simulink model "RL_sus_quarter_sim"  (R2025a)
settings: Solver=FixedStepAuto  StartTime=0.0  StopTime=20  FixedStep=0.001  RelTol=1e-3
model workspace (MAT data in the model file):
  G0 : Simulink.Parameter (value not decoded)
  Q_F : Simulink.Parameter (value not decoded)
  Q_dot_s : Simulink.Parameter (value not decoded)
  Q_dot_s_h : Simulink.Parameter (value not decoded)
  Q_dot_u : Simulink.Parameter (value not decoded)
  Q_flec : Simulink.Parameter (value not decoded)
  Q_flec_t : Simulink.Parameter (value not decoded)
  b_deflec : Simulink.Parameter (value not decoded)
  bump_height : Simulink.Parameter (value not decoded)
  bump_lenth : Simulink.Parameter (value not decoded)
  bump_start : Simulink.Parameter (value not decoded)
  f0 : Simulink.Parameter (value not decoded)
  kt : Simulink.Parameter (value not decoded)
  ms : Simulink.Parameter (value not decoded)
  n0 : Simulink.Parameter (value not decoded)
  n1 : Simulink.Parameter (value not decoded)
  omega_1 : Simulink.Parameter (value not decoded)
  omega_2 : Simulink.Parameter (value not decoded)
  omega_3 : Simulink.Parameter (value not decoded)
  omega_4 : Simulink.Parameter (value not decoded)
  ramp_height : Simulink.Parameter (value not decoded)
  ramp_lenth : Simulink.Parameter (value not decoded)
  ramp_start : Simulink.Parameter (value not decoded)
  sine_amp : Simulink.Parameter (value not decoded)
  sine_freq : Simulink.Parameter (value not decoded)
  u : Simulink.Parameter (value not decoded)
symbols that are objects in the model workspace (value not decoded): b_deflec, bump_height, bump_lenth, bump_start, f0, G0, kt, ms, n0, n1, omega_1, omega_2, omega_3, omega_4, Q_dot_s, Q_dot_s_h, Q_F, Q_flec, Q_flec_t, ramp_height, ramp_lenth, ramp_start, sine_amp, sine_freq
undefined symbols (not defined in the file): Ground, Hook, SH_ADD_new_as_as_xdef
libraries: fl_lib x250, nesl_utility x48, sharedTrackingLibrary x34, dspstat3 x18, simulink x3, deeplib x2, slpidlib x1
(part 10 of 12)

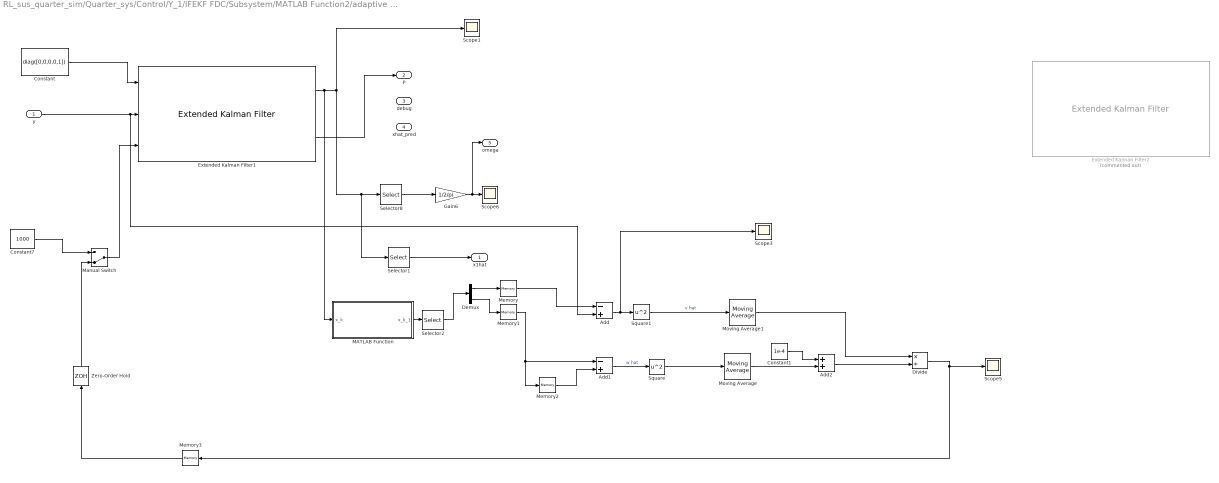
== system RL_sus_quarter_sim/Quarter_sys/Control/Y_1/IFEKF FDC/Subsystem/MATLAB Function2/adaptive IFEKF simple ==
  y : Inport
  Add : Sum  Inputs=-+
  Add1 : Sum  Inputs=-+
  Add2 : Sum
  Constant : Constant  Value=diag([0,0,0,0,1])
  Constant1 : Constant  Value=1e-4
  Constant7 : Constant  Value=1000  SampleTime=0.001
  Demux : Demux  Outputs=2
  Divide : Product  Inputs=*/
  Extended Kalman Filter1 : sharedTrackingLibrary/Extended Kalman Filter  StateTransitionFcn=IFEKF_tfcn_simp  HasStateTransitionJacobianFcn=on  StateTransitionJacobianFcn=IFEKF_jcob_fcn_simp  HasAdditiveProcessNoise=Additive  ProcessNoise=[0,0,1e-7,1e-10,0]  HasTimeVaryingProcessNoise=on  HasStateTransitionFcnExtraArgument=0  InitialState=[0;-1;0;-1;10*2*pi;]  InitialStateCovariance=[1e-1,1e-1,1e-1,1e-1,1e-5]  MeasurementFcn1=IFEKF_measure_fcn_simp  HasMeasurementJacobianFcn1=on  MeasurementJacobianFcn1=IFEKF_mea_jcob_fcn_simp  HasMeasurementEnablePort1=off  HasAdditiveMeasurementNoise1=Additive  MeasurementNoise1=0.0001  HasTimeVaryingMeasurementNoise1=on  HasMeasurementFcnExtraArgument1=0  HasMeasurementWrapping1=off  MeasurementFcn2=myMeasurementFcn  HasMeasurementJacobianFcn2=off  HasMeasurementEnablePort2=off  HasAdditiveMeasurementNoise2=Additive  MeasurementNoise2=1  HasTimeVaryingMeasurementNoise2=off  HasMeasurementFcnExtraArgument2=0  HasMeasurementWrapping2=off  MeasurementFcn3=myMeasurementFcn  HasMeasurementJacobianFcn3=off  HasMeasurementEnablePort3=off  HasAdditiveMeasurementNoise3=Additive  MeasurementNoise3=1  HasTimeVaryingMeasurementNoise3=off  HasMeasurementFcnExtraArgument3=0  HasMeasurementWrapping3=off  MeasurementFcn4=myMeasurementFcn  HasMeasurementJacobianFcn4=off  HasMeasurementEnablePort4=off  HasAdditiveMeasurementNoise4=Additive  MeasurementNoise4=1  HasTimeVaryingMeasurementNoise4=off  HasMeasurementFcnExtraArgument4=0  HasMeasurementWrapping4=off  MeasurementFcn5=myMeasurementFcn  HasMeasurementJacobianFcn5=off  HasMeasurementEnablePort5=off  HasAdditiveMeasurementNoise5=Additive  MeasurementNoise5=1  HasTimeVaryingMeasurementNoise5=off  HasMeasurementFcnExtraArgument5=0  HasMeasurementWrapping5=off  EnableMultirate=off  StateTransitionFcnSampleTime=1  MeasurementFcn1SampleTime=1  MeasurementFcn2SampleTime=1  MeasurementFcn3SampleTime=1  MeasurementFcn4SampleTime=1  MeasurementFcn5SampleTime=1  UseCurrentEstimator=off  OutputStateCovariance=on  DataType=double  SampleTime=0.001  NumberOfMeasurements=1
  Extended Kalman Filter2 : sharedTrackingLibrary/Extended Kalman Filter  Commented=on  StateTransitionFcn=IFEKF_tfcn_simp  HasStateTransitionJacobianFcn=on  StateTransitionJacobianFcn=IFEKF_jcob_fcn_simp  HasAdditiveProcessNoise=Additive  ProcessNoise=[0,0,1e-7,1e-10,0]  HasTimeVaryingProcessNoise=on  HasStateTransitionFcnExtraArgument=0  InitialState=[0;-1;0;-1;8*2*pi;]  InitialStateCovariance=[1e-1,1e-1,1e-1,1e-1,1e-5]  MeasurementFcn1=IFEKF_measure_fcn_simp  HasMeasurementJacobianFcn1=on  MeasurementJacobianFcn1=IFEKF_mea_jcob_fcn_simp  HasMeasurementEnablePort1=off  HasAdditiveMeasurementNoise1=Additive  MeasurementNoise1=0.0001  HasTimeVaryingMeasurementNoise1=on  HasMeasurementFcnExtraArgument1=0  HasMeasurementWrapping1=off  MeasurementFcn2=myMeasurementFcn  HasMeasurementJacobianFcn2=off  HasMeasurementEnablePort2=off  HasAdditiveMeasurementNoise2=Additive  MeasurementNoise2=1  HasTimeVaryingMeasurementNoise2=off  HasMeasurementFcnExtraArgument2=0  HasMeasurementWrapping2=off  MeasurementFcn3=myMeasurementFcn  HasMeasurementJacobianFcn3=off  HasMeasurementEnablePort3=off  HasAdditiveMeasurementNoise3=Additive  MeasurementNoise3=1  HasTimeVaryingMeasurementNoise3=off  HasMeasurementFcnExtraArgument3=0  HasMeasurementWrapping3=off  MeasurementFcn4=myMeasurementFcn  HasMeasurementJacobianFcn4=off  HasMeasurementEnablePort4=off  HasAdditiveMeasurementNoise4=Additive  MeasurementNoise4=1  HasTimeVaryingMeasurementNoise4=off  HasMeasurementFcnExtraArgument4=0  HasMeasurementWrapping4=off  MeasurementFcn5=myMeasurementFcn  HasMeasurementJacobianFcn5=off  HasMeasurementEnablePort5=off  HasAdditiveMeasurementNoise5=Additive  MeasurementNoise5=1  HasTimeVaryingMeasurementNoise5=off  HasMeasurementFcnExtraArgument5=0  HasMeasurementWrapping5=off  EnableMultirate=off  StateTransitionFcnSampleTime=1  MeasurementFcn1SampleTime=1  MeasurementFcn2SampleTime=1  MeasurementFcn3SampleTime=1  MeasurementFcn4SampleTime=1  MeasurementFcn5SampleTime=1  UseCurrentEstimator=off  OutputStateCovariance=on  DataType=double  SampleTime=0.001  NumberOfMeasurements=1
  Gain6 : Gain  Gain=1/2/pi
  MATLAB Function : MATLAB Function  TreatAsAtomicUnit=on
  Manual Switch : ManualSwitch  CurrentSetting=0
  Memory : Memory
  Memory1 : Memory  InitialCondition=2
  Memory2 : Memory  InitialCondition=1
  Memory3 : Memory  InitialCondition=10
  Moving Average : dspstat3/Moving Average  Method=Exponential weighting  ForgettingFactorPort=off  SpecifyWindowLength=off  WindowLength=100  OverlapLength=50  AllowArbitraryInputLength=on  ForgettingFactor=0.999  SimulateUsing=Interpreted execution
  Moving Average1 : dspstat3/Moving Average  Method=Exponential weighting  ForgettingFactorPort=off  SpecifyWindowLength=off  WindowLength=100  OverlapLength=50  AllowArbitraryInputLength=on  ForgettingFactor=0.995  SimulateUsing=Interpreted execution
  Scope{1,3,5..6} (4 alike) : Scope
      Scope1 settings: ActiveDisplayYMinimum=-543.51762  ActiveDisplayYMaximum=583.84894  DataLoggingVariableName=ScopeData3
      Scope3 settings: ActiveDisplayYMinimum=-2.16466  ActiveDisplayYMaximum=0.26631  DataLoggingVariableName=ScopeData4
      Scope5 settings: ActiveDisplayYMinimum=-0.0003  ActiveDisplayYMaximum=0.00266  DataLoggingVariableName=ScopeData6
      Scope6 settings: ActiveDisplayYMinimum=5.69068  ActiveDisplayYMaximum=19.94579  DataLoggingVariableName=ScopeData8
  Selector1 : Selector  InputPortWidth=5  IndexOptions=Index vector (dialog)  Indices=[1]  OutputSizes=1
  Selector2 : Selector  InputPortWidth=5  IndexOptions=Index vector (dialog)  Indices=[1 5]  OutputSizes=1
  Selector8 : Selector  InputPortWidth=5  IndexOptions=Index vector (dialog)  Indices=[5]  OutputSizes=1
  Square : Math  Operator=square
  Square1 : Math  Operator=square
  Zero-Order Hold : ZeroOrderHold  SampleTime=0.001
  x1hat : Outport
  P : Outport  Port=2
  debug : Outport  Port=3
  xhat_pred : Outport  Port=4
  omega : Outport  Port=5
  wires:
  Add1/1 -> Square/1  "w hat"
  Demux/2 -> Memory1/1
  Constant1/1 -> Add2/1
  Zero-Order Hold/1 -> Manual Switch/2
  Memory2/1 -> Add1/2
  Manual Switch/1 -> Extended Kalman Filter1/3
  MATLAB Function/1(x_k_1) -> Selector2/1
  Moving Average1/1 -> Divide/1
  Selector2/1 -> Demux/1
  Add2/1 -> Divide/2
  Constant/1 -> Extended Kalman Filter1/1
  Selector1/1 -> x1hat/1
  Moving Average/1 -> Add2/2
  Memory/1 -> Add/1
  Extended Kalman Filter1/1 -> MATLAB Function/1(x_k), Scope1/1, Selector8/1, Selector1/1
  y/1 -> Add/2, Extended Kalman Filter1/2
  Memory1/1 -> Add1/1, Memory2/1
  Square/1 -> Moving Average/1
  Square1/1 -> Moving Average1/1  "v hat"
  Extended Kalman Filter1/2 -> P/1
  Divide/1 -> Memory3/1, Scope5/1
  Selector8/1 -> Gain6/1
  Demux/1 -> Memory/1
  Add/1 -> Scope3/1, Square1/1
  Memory3/1 -> Zero-Order Hold/1
  Gain6/1 -> Scope6/1, omega/1
  Constant7/1 -> Manual Switch/1

== system RL_sus_quarter_sim/Quarter_sys/Control/Y_1/IFEKF SHADD/Subsystem/MATLAB Function2/EKF epsilon ==
  y : Inport
  epsilon : Inport  Port=2
  Constant : Constant  Value=diag([0,0,1,0])
  Constant7 : Constant  Value=500  SampleTime=0.001
  Extended Kalman Filter1 : sharedTrackingLibrary/Extended Kalman Filter  StateTransitionFcn=IFEKF_tfcn_ep  HasStateTransitionJacobianFcn=on  StateTransitionJacobianFcn=IFEKF_jcob_fcn_ep  HasAdditiveProcessNoise=Additive  ProcessNoise=[0,0,1e-7,1e-10]  HasTimeVaryingProcessNoise=on  HasStateTransitionFcnExtraArgument=1  InitialState=[0;-0.2;1*2*pi;0.2;]  InitialStateCovariance=[1e-1,1e-1,1e-1,1e-5]  MeasurementFcn1=IFEKF_measure_fcn_mod  HasMeasurementJacobianFcn1=on  MeasurementJacobianFcn1=IFEKF_mea_jcob_fcn_mod  HasMeasurementEnablePort1=off  HasAdditiveMeasurementNoise1=Additive  MeasurementNoise1=0.0001  HasTimeVaryingMeasurementNoise1=on  HasMeasurementFcnExtraArgument1=0  HasMeasurementWrapping1=off  MeasurementFcn2=myMeasurementFcn  HasMeasurementJacobianFcn2=off  HasMeasurementEnablePort2=off  HasAdditiveMeasurementNoise2=Additive  MeasurementNoise2=1  HasTimeVaryingMeasurementNoise2=off  HasMeasurementFcnExtraArgument2=0  HasMeasurementWrapping2=off  MeasurementFcn3=myMeasurementFcn  HasMeasurementJacobianFcn3=off  HasMeasurementEnablePort3=off  HasAdditiveMeasurementNoise3=Additive  MeasurementNoise3=1  HasTimeVaryingMeasurementNoise3=off  HasMeasurementFcnExtraArgument3=0  HasMeasurementWrapping3=off  MeasurementFcn4=myMeasurementFcn  HasMeasurementJacobianFcn4=off  HasMeasurementEnablePort4=off  HasAdditiveMeasurementNoise4=Additive  MeasurementNoise4=1  HasTimeVaryingMeasurementNoise4=off  HasMeasurementFcnExtraArgument4=0  HasMeasurementWrapping4=off  MeasurementFcn5=myMeasurementFcn  HasMeasurementJacobianFcn5=off  HasMeasurementEnablePort5=off  HasAdditiveMeasurementNoise5=Additive  MeasurementNoise5=1  HasTimeVaryingMeasurementNoise5=off  HasMeasurementFcnExtraArgument5=0  HasMeasurementWrapping5=off  EnableMultirate=off  StateTransitionFcnSampleTime=1  MeasurementFcn1SampleTime=1  MeasurementFcn2SampleTime=1  MeasurementFcn3SampleTime=1  MeasurementFcn4SampleTime=1  MeasurementFcn5SampleTime=1  UseCurrentEstimator=off  OutputStateCovariance=on  DataType=double  SampleTime=0.001  NumberOfMeasurements=1
  Gain6 : Gain  Gain=1/2/pi
  Scope6 : Scope
      settings: ActiveDisplayYMinimum=-0.3996  ActiveDisplayYMaximum=6.53697  DataLoggingVariableName=ScopeData2
  Selector1 : Selector  InputPortWidth=4  IndexOptions=Index vector (dialog)  Indices=[1]  OutputSizes=1
  Selector8 : Selector  InputPortWidth=4  IndexOptions=Index vector (dialog)  Indices=[3]  OutputSizes=1
  x1hat : Outport
  P : Outport  Port=2
  debug : Outport  Port=3
  xhat_pred : Outport  Port=4
  y_residual : Outport  Port=5
  omega : Outport  Port=6
  wires:
  Selector1/1 -> x1hat/1
  Extended Kalman Filter1/1 -> Selector8/1, Selector1/1
  Selector8/1 -> Gain6/1
  Gain6/1 -> Scope6/1, omega/1
  Constant/1 -> Extended Kalman Filter1/1
  epsilon/1 -> Extended Kalman Filter1/2
  Constant7/1 -> Extended Kalman Filter1/4
  Extended Kalman Filter1/2 -> P/1
  y/1 -> Extended Kalman Filter1/3

== system RL_sus_quarter_sim/Quarter_sys/Control/Y_1/IFEKF SHADD/Subsystem/MATLAB Function2/EKF simple Amp ==
  y : Inport
  epsilon : Inport  Port=2
  Constant5 : Constant  Value=0.1e-5
  Constant7 : Constant  Value=0.11  SampleTime=0.001
  Extended Kalman Filter1 : sharedTrackingLibrary/Extended Kalman Filter  StateTransitionFcn=IFEKF_tfcn_amp  HasStateTransitionJacobianFcn=on  StateTransitionJacobianFcn=IFEKF_jcob_fcn_amp  HasAdditiveProcessNoise=Additive  ProcessNoise=[0,0,1e-7,1e-10]  HasTimeVaryingProcessNoise=on  HasStateTransitionFcnExtraArgument=1  InitialState=[0;-0.5;2*pi;0.5;]  InitialStateCovariance=[1e-1,1e-1,1e-1,1e-5]  MeasurementFcn1=IFEKF_measure_fcn_amp  HasMeasurementJacobianFcn1=on  MeasurementJacobianFcn1=IFEKF_mea_jcob_fcn_amp  HasMeasurementEnablePort1=off  HasAdditiveMeasurementNoise1=Additive  MeasurementNoise1=0.0001  HasTimeVaryingMeasurementNoise1=on  HasMeasurementFcnExtraArgument1=0  HasMeasurementWrapping1=off  MeasurementFcn2=myMeasurementFcn  HasMeasurementJacobianFcn2=off  HasMeasurementEnablePort2=off  HasAdditiveMeasurementNoise2=Additive  MeasurementNoise2=1  HasTimeVaryingMeasurementNoise2=off  HasMeasurementFcnExtraArgument2=0  HasMeasurementWrapping2=off  MeasurementFcn3=myMeasurementFcn  HasMeasurementJacobianFcn3=off  HasMeasurementEnablePort3=off  HasAdditiveMeasurementNoise3=Additive  MeasurementNoise3=1  HasTimeVaryingMeasurementNoise3=off  HasMeasurementFcnExtraArgument3=0  HasMeasurementWrapping3=off  MeasurementFcn4=myMeasurementFcn  HasMeasurementJacobianFcn4=off  HasMeasurementEnablePort4=off  HasAdditiveMeasurementNoise4=Additive  MeasurementNoise4=1  HasTimeVaryingMeasurementNoise4=off  HasMeasurementFcnExtraArgument4=0  HasMeasurementWrapping4=off  MeasurementFcn5=myMeasurementFcn  HasMeasurementJacobianFcn5=off  HasMeasurementEnablePort5=off  HasAdditiveMeasurementNoise5=Additive  MeasurementNoise5=1  HasTimeVaryingMeasurementNoise5=off  HasMeasurementFcnExtraArgument5=0  HasMeasurementWrapping5=off  EnableMultirate=off  StateTransitionFcnSampleTime=1  MeasurementFcn1SampleTime=1  MeasurementFcn2SampleTime=1  MeasurementFcn3SampleTime=1  MeasurementFcn4SampleTime=1  MeasurementFcn5SampleTime=1  UseCurrentEstimator=off  OutputStateCovariance=on  DataType=double  SampleTime=0.001  NumberOfMeasurements=1
  Gain6 : Gain  Gain=1/2/pi
  MATLAB Function : MATLAB Function
  Scope1 : Scope
      settings: ActiveDisplayYMinimum=-1.3479  ActiveDisplayYMaximum=7.13108  DataLoggingVariableName=ScopeData7
  Scope6 : Scope
      settings: ActiveDisplayYMinimum=0.9999988  ActiveDisplayYMaximum=1.0000001
  Selector1 : Selector  InputPortWidth=4  IndexOptions=Index vector (dialog)  Indices=[1]  OutputSizes=1
  Selector8 : Selector  InputPortWidth=4  IndexOptions=Index vector (dialog)  Indices=[3]  OutputSizes=1
  x1hat : Outport
  P : Outport  Port=2
  debug : Outport  Port=3
  xhat_pred : Outport  Port=4
  y_residual : Outport  Port=5
  omega : Outport  Port=6
  wires:
  Selector1/1 -> x1hat/1
  Gain6/1 -> Scope6/1, omega/1
  Selector8/1 -> Gain6/1
  Extended Kalman Filter1/1 -> Scope1/1, Selector8/1, Selector1/1
  MATLAB Function/1(y) -> Extended Kalman Filter1/1
  y/1 -> Extended Kalman Filter1/3
  Extended Kalman Filter1/2 -> P/1
  Constant5/1 -> MATLAB Function/1(gamma)
  Constant7/1 -> Extended Kalman Filter1/4
  epsilon/1 -> Extended Kalman Filter1/2

== system RL_sus_quarter_sim/Quarter_sys/Control/Y_1/IFEKF SHADD/Subsystem/MATLAB Function2/IFEKF simple ==
  y : Inport
  Constant : Constant  Value=diag([0,0,0,0,1])
  Constant7 : Constant  Value=10  SampleTime=0.001
  Extended Kalman Filter1 : sharedTrackingLibrary/Extended Kalman Filter  StateTransitionFcn=IFEKF_tfcn_simp  HasStateTransitionJacobianFcn=on  StateTransitionJacobianFcn=IFEKF_jcob_fcn_simp  HasAdditiveProcessNoise=Additive  ProcessNoise=[0,0,1e-7,1e-10,0]  HasTimeVaryingProcessNoise=on  HasStateTransitionFcnExtraArgument=0  InitialState=[0;-1;0;-1;0.1*pi;]  InitialStateCovariance=[1e-1,1e-1,1e-1,1e-1,1e-5]  MeasurementFcn1=IFEKF_measure_fcn_simp  HasMeasurementJacobianFcn1=on  MeasurementJacobianFcn1=IFEKF_mea_jcob_fcn_simp  HasMeasurementEnablePort1=off  HasAdditiveMeasurementNoise1=Additive  MeasurementNoise1=0.0001  HasTimeVaryingMeasurementNoise1=on  HasMeasurementFcnExtraArgument1=0  HasMeasurementWrapping1=off  MeasurementFcn2=myMeasurementFcn  HasMeasurementJacobianFcn2=off  HasMeasurementEnablePort2=off  HasAdditiveMeasurementNoise2=Additive  MeasurementNoise2=1  HasTimeVaryingMeasurementNoise2=off  HasMeasurementFcnExtraArgument2=0  HasMeasurementWrapping2=off  MeasurementFcn3=myMeasurementFcn  HasMeasurementJacobianFcn3=off  HasMeasurementEnablePort3=off  HasAdditiveMeasurementNoise3=Additive  MeasurementNoise3=1  HasTimeVaryingMeasurementNoise3=off  HasMeasurementFcnExtraArgument3=0  HasMeasurementWrapping3=off  MeasurementFcn4=myMeasurementFcn  HasMeasurementJacobianFcn4=off  HasMeasurementEnablePort4=off  HasAdditiveMeasurementNoise4=Additive  MeasurementNoise4=1  HasTimeVaryingMeasurementNoise4=off  HasMeasurementFcnExtraArgument4=0  HasMeasurementWrapping4=off  MeasurementFcn5=myMeasurementFcn  HasMeasurementJacobianFcn5=off  HasMeasurementEnablePort5=off  HasAdditiveMeasurementNoise5=Additive  MeasurementNoise5=1  HasTimeVaryingMeasurementNoise5=off  HasMeasurementFcnExtraArgument5=0  HasMeasurementWrapping5=off  EnableMultirate=off  StateTransitionFcnSampleTime=1  MeasurementFcn1SampleTime=1  MeasurementFcn2SampleTime=1  MeasurementFcn3SampleTime=1  MeasurementFcn4SampleTime=1  MeasurementFcn5SampleTime=1  UseCurrentEstimator=off  OutputStateCovariance=on  DataType=double  SampleTime=0.001  NumberOfMeasurements=1
  Gain6 : Gain  Gain=1/2/pi
  Scope1 : Scope
      settings: ActiveDisplayYMinimum=-108223.31295  ActiveDisplayYMaximum=120159.3313  DataLoggingVariableName=ScopeData2
  Scope6 : Scope
      settings: ActiveDisplayYMinimum=-5.04517  ActiveDisplayYMaximum=3.95687  DataLoggingVariableName=ScopeData3
  Selector1 : Selector  InputPortWidth=5  IndexOptions=Index vector (dialog)  Indices=[1]  OutputSizes=1
  Selector8 : Selector  InputPortWidth=5  IndexOptions=Index vector (dialog)  Indices=[5]  OutputSizes=1
  x1hat : Outport
  P : Outport  Port=2
  debug : Outport  Port=3
  xhat_pred : Outport  Port=4
  y_residual : Outport  Port=5
  omega : Outport  Port=6
  wires:
  Extended Kalman Filter1/1 -> Scope1/1, Selector8/1, Selector1/1
  Selector1/1 -> x1hat/1
  Selector8/1 -> Gain6/1
  Gain6/1 -> Scope6/1, omega/1
  Constant/1 -> Extended Kalman Filter1/1
  Constant7/1 -> Extended Kalman Filter1/3
  Extended Kalman Filter1/2 -> P/1
  y/1 -> Extended Kalman Filter1/2

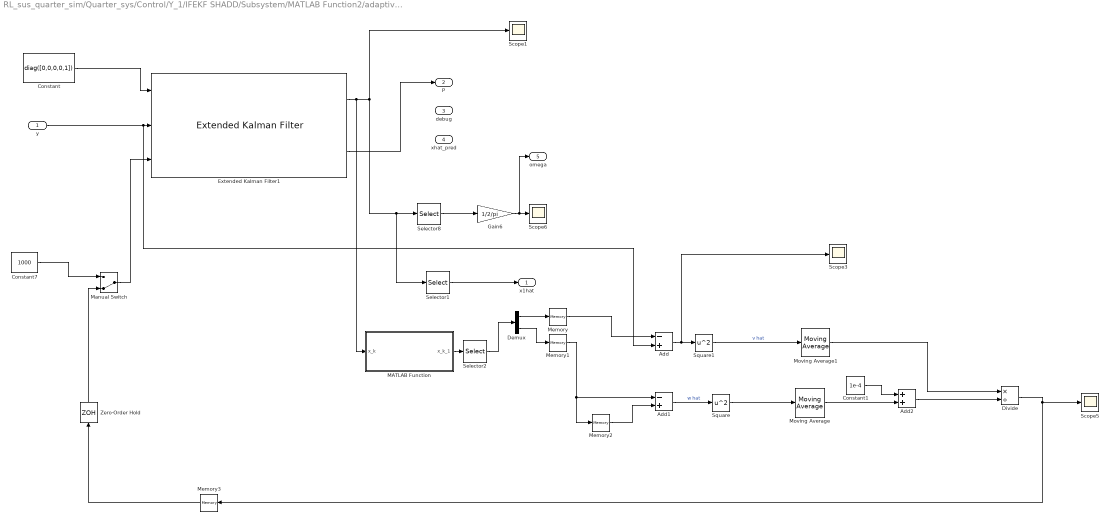
== system RL_sus_quarter_sim/Quarter_sys/Control/Y_1/IFEKF SHADD/Subsystem/MATLAB Function2/adaptive IFEKF simple ==
  y : Inport
  Add : Sum  Inputs=-+
  Add1 : Sum  Inputs=-+
  Add2 : Sum
  Constant : Constant  Value=diag([0,0,0,0,1])
  Constant1 : Constant  Value=1e-4
  Constant7 : Constant  Value=1000  SampleTime=0.001
  Demux : Demux  Outputs=2
  Divide : Product  Inputs=*/
  Extended Kalman Filter1 : sharedTrackingLibrary/Extended Kalman Filter  StateTransitionFcn=IFEKF_tfcn_simp  HasStateTransitionJacobianFcn=on  StateTransitionJacobianFcn=IFEKF_jcob_fcn_simp  HasAdditiveProcessNoise=Additive  ProcessNoise=[0,0,1e-7,1e-10,0]  HasTimeVaryingProcessNoise=on  HasStateTransitionFcnExtraArgument=0  InitialState=[0;-1;0;-1;0.1*pi;]  InitialStateCovariance=[1e-1,1e-1,1e-1,1e-1,1e-5]  MeasurementFcn1=IFEKF_measure_fcn_simp  HasMeasurementJacobianFcn1=on  MeasurementJacobianFcn1=IFEKF_mea_jcob_fcn_simp  HasMeasurementEnablePort1=off  HasAdditiveMeasurementNoise1=Additive  MeasurementNoise1=0.0001  HasTimeVaryingMeasurementNoise1=on  HasMeasurementFcnExtraArgument1=0  HasMeasurementWrapping1=off  MeasurementFcn2=myMeasurementFcn  HasMeasurementJacobianFcn2=off  HasMeasurementEnablePort2=off  HasAdditiveMeasurementNoise2=Additive  MeasurementNoise2=1  HasTimeVaryingMeasurementNoise2=off  HasMeasurementFcnExtraArgument2=0  HasMeasurementWrapping2=off  MeasurementFcn3=myMeasurementFcn  HasMeasurementJacobianFcn3=off  HasMeasurementEnablePort3=off  HasAdditiveMeasurementNoise3=Additive  MeasurementNoise3=1  HasTimeVaryingMeasurementNoise3=off  HasMeasurementFcnExtraArgument3=0  HasMeasurementWrapping3=off  MeasurementFcn4=myMeasurementFcn  HasMeasurementJacobianFcn4=off  HasMeasurementEnablePort4=off  HasAdditiveMeasurementNoise4=Additive  MeasurementNoise4=1  HasTimeVaryingMeasurementNoise4=off  HasMeasurementFcnExtraArgument4=0  HasMeasurementWrapping4=off  MeasurementFcn5=myMeasurementFcn  HasMeasurementJacobianFcn5=off  HasMeasurementEnablePort5=off  HasAdditiveMeasurementNoise5=Additive  MeasurementNoise5=1  HasTimeVaryingMeasurementNoise5=off  HasMeasurementFcnExtraArgument5=0  HasMeasurementWrapping5=off  EnableMultirate=off  StateTransitionFcnSampleTime=1  MeasurementFcn1SampleTime=1  MeasurementFcn2SampleTime=1  MeasurementFcn3SampleTime=1  MeasurementFcn4SampleTime=1  MeasurementFcn5SampleTime=1  UseCurrentEstimator=off  OutputStateCovariance=on  DataType=double  SampleTime=0.001  NumberOfMeasurements=1
  Gain6 : Gain  Gain=1/2/pi
  MATLAB Function : MATLAB Function  TreatAsAtomicUnit=on
  Manual Switch : ManualSwitch  CurrentSetting=0
  Memory : Memory  InitialCondition=5
  Memory1 : Memory
  Memory2 : Memory  InitialCondition=1
  Memory3 : Memory  InitialCondition=10
  Moving Average : dspstat3/Moving Average  Method=Exponential weighting  ForgettingFactorPort=off  SpecifyWindowLength=off  WindowLength=100  OverlapLength=50  AllowArbitraryInputLength=on  ForgettingFactor=0.999  SimulateUsing=Interpreted execution
  Moving Average1 : dspstat3/Moving Average  Method=Exponential weighting  ForgettingFactorPort=off  SpecifyWindowLength=off  WindowLength=100  OverlapLength=50  AllowArbitraryInputLength=on  ForgettingFactor=0.999  SimulateUsing=Interpreted execution
  Scope{1,3,5..6} (4 alike) : Scope
      Scope1 settings: ActiveDisplayYMinimum=-108223.31295  ActiveDisplayYMaximum=120159.3313  DataLoggingVariableName=ScopeData3
      Scope3 settings: ActiveDisplayYMinimum=-5.93217  ActiveDisplayYMaximum=3.44712  DataLoggingVariableName=ScopeData4
      Scope5 settings: ActiveDisplayYMinimum=-180.87615  ActiveDisplayYMaximum=1627.8871  DataLoggingVariableName=ScopeData6
      Scope6 settings: ActiveDisplayYMinimum=-2.71822  ActiveDisplayYMaximum=5.24485  DataLoggingVariableName=ScopeData8
  Selector1 : Selector  InputPortWidth=5  IndexOptions=Index vector (dialog)  Indices=[1]  OutputSizes=1
  Selector2 : Selector  InputPortWidth=5  IndexOptions=Index vector (dialog)  Indices=[1 5]  OutputSizes=1
  Selector8 : Selector  InputPortWidth=5  IndexOptions=Index vector (dialog)  Indices=[5]  OutputSizes=1
  Square : Math  Operator=square
  Square1 : Math  Operator=square
  Zero-Order Hold : ZeroOrderHold  SampleTime=0.001
  x1hat : Outport
  P : Outport  Port=2
  debug : Outport  Port=3
  xhat_pred : Outport  Port=4
  omega : Outport  Port=5
  wires:
  Constant7/1 -> Manual Switch/1
  Gain6/1 -> omega/1, Scope6/1
  Memory3/1 -> Zero-Order Hold/1
  Add/1 -> Square1/1, Scope3/1
  Demux/1 -> Memory/1
  Selector8/1 -> Gain6/1
  Divide/1 -> Scope5/1, Memory3/1
  Extended Kalman Filter1/2 -> P/1
  Square1/1 -> Moving Average1/1  "v hat"
  Square/1 -> Moving Average/1
  Memory1/1 -> Memory2/1, Add1/1
  y/1 -> Extended Kalman Filter1/2, Add/2
  Extended Kalman Filter1/1 -> Selector1/1, Selector8/1, Scope1/1, MATLAB Function/1(x_k)
  Memory/1 -> Add/1
  Moving Average/1 -> Add2/2
  Selector1/1 -> x1hat/1
  Constant/1 -> Extended Kalman Filter1/1
  Add2/1 -> Divide/2
  Selector2/1 -> Demux/1
  Moving Average1/1 -> Divide/1
  MATLAB Function/1(x_k_1) -> Selector2/1
  Manual Switch/1 -> Extended Kalman Filter1/3
  Memory2/1 -> Add1/2
  Zero-Order Hold/1 -> Manual Switch/2
  Constant1/1 -> Add2/1
  Demux/2 -> Memory1/1
  Add1/1 -> Square/1  "w hat"

== system RL_sus_quarter_sim/Quarter_sys/Control/Y_1/IFEKF Select c/Subsystem/MATLAB Function2/EKF epsilon ==
  y : Inport
  epsilon : Inport  Port=2
  Constant : Constant  Value=diag([0,0,1,0])
  Constant7 : Constant  Value=500  SampleTime=0.001
  Extended Kalman Filter1 : sharedTrackingLibrary/Extended Kalman Filter  StateTransitionFcn=IFEKF_tfcn_ep  HasStateTransitionJacobianFcn=on  StateTransitionJacobianFcn=IFEKF_jcob_fcn_ep  HasAdditiveProcessNoise=Additive  ProcessNoise=[0,0,1e-7,1e-10]  HasTimeVaryingProcessNoise=on  HasStateTransitionFcnExtraArgument=1  InitialState=[0;-0.2;1*2*pi;0.2;]  InitialStateCovariance=[1e-1,1e-1,1e-1,1e-5]  MeasurementFcn1=IFEKF_measure_fcn_mod  HasMeasurementJacobianFcn1=on  MeasurementJacobianFcn1=IFEKF_mea_jcob_fcn_mod  HasMeasurementEnablePort1=off  HasAdditiveMeasurementNoise1=Additive  MeasurementNoise1=0.0001  HasTimeVaryingMeasurementNoise1=on  HasMeasurementFcnExtraArgument1=0  HasMeasurementWrapping1=off  MeasurementFcn2=myMeasurementFcn  HasMeasurementJacobianFcn2=off  HasMeasurementEnablePort2=off  HasAdditiveMeasurementNoise2=Additive  MeasurementNoise2=1  HasTimeVaryingMeasurementNoise2=off  HasMeasurementFcnExtraArgument2=0  HasMeasurementWrapping2=off  MeasurementFcn3=myMeasurementFcn  HasMeasurementJacobianFcn3=off  HasMeasurementEnablePort3=off  HasAdditiveMeasurementNoise3=Additive  MeasurementNoise3=1  HasTimeVaryingMeasurementNoise3=off  HasMeasurementFcnExtraArgument3=0  HasMeasurementWrapping3=off  MeasurementFcn4=myMeasurementFcn  HasMeasurementJacobianFcn4=off  HasMeasurementEnablePort4=off  HasAdditiveMeasurementNoise4=Additive  MeasurementNoise4=1  HasTimeVaryingMeasurementNoise4=off  HasMeasurementFcnExtraArgument4=0  HasMeasurementWrapping4=off  MeasurementFcn5=myMeasurementFcn  HasMeasurementJacobianFcn5=off  HasMeasurementEnablePort5=off  HasAdditiveMeasurementNoise5=Additive  MeasurementNoise5=1  HasTimeVaryingMeasurementNoise5=off  HasMeasurementFcnExtraArgument5=0  HasMeasurementWrapping5=off  EnableMultirate=off  StateTransitionFcnSampleTime=1  MeasurementFcn1SampleTime=1  MeasurementFcn2SampleTime=1  MeasurementFcn3SampleTime=1  MeasurementFcn4SampleTime=1  MeasurementFcn5SampleTime=1  UseCurrentEstimator=off  OutputStateCovariance=on  DataType=double  SampleTime=0.001  NumberOfMeasurements=1
  Gain6 : Gain  Gain=1/2/pi
  Scope6 : Scope
      settings: ActiveDisplayYMinimum=-0.3996  ActiveDisplayYMaximum=6.53697  DataLoggingVariableName=ScopeData2
  Selector1 : Selector  InputPortWidth=4  IndexOptions=Index vector (dialog)  Indices=[1]  OutputSizes=1
  Selector8 : Selector  InputPortWidth=4  IndexOptions=Index vector (dialog)  Indices=[3]  OutputSizes=1
  x1hat : Outport
  P : Outport  Port=2
  debug : Outport  Port=3
  xhat_pred : Outport  Port=4
  y_residual : Outport  Port=5
  omega : Outport  Port=6
  wires:
  y/1 -> Extended Kalman Filter1/3
  Extended Kalman Filter1/2 -> P/1
  Constant7/1 -> Extended Kalman Filter1/4
  epsilon/1 -> Extended Kalman Filter1/2
  Constant/1 -> Extended Kalman Filter1/1
  Gain6/1 -> omega/1, Scope6/1
  Selector8/1 -> Gain6/1
  Extended Kalman Filter1/1 -> Selector1/1, Selector8/1
  Selector1/1 -> x1hat/1

== system RL_sus_quarter_sim/Quarter_sys/Control/Y_1/IFEKF Select c/Subsystem/MATLAB Function2/EKF simple Amp ==
  y : Inport
  epsilon : Inport  Port=2
  Constant5 : Constant  Value=0.1e-5
  Constant7 : Constant  Value=0.11  SampleTime=0.001
  Extended Kalman Filter1 : sharedTrackingLibrary/Extended Kalman Filter  StateTransitionFcn=IFEKF_tfcn_amp  HasStateTransitionJacobianFcn=on  StateTransitionJacobianFcn=IFEKF_jcob_fcn_amp  HasAdditiveProcessNoise=Additive  ProcessNoise=[0,0,1e-7,1e-10]  HasTimeVaryingProcessNoise=on  HasStateTransitionFcnExtraArgument=1  InitialState=[0;-0.5;2*pi;0.5;]  InitialStateCovariance=[1e-1,1e-1,1e-1,1e-5]  MeasurementFcn1=IFEKF_measure_fcn_amp  HasMeasurementJacobianFcn1=on  MeasurementJacobianFcn1=IFEKF_mea_jcob_fcn_amp  HasMeasurementEnablePort1=off  HasAdditiveMeasurementNoise1=Additive  MeasurementNoise1=0.0001  HasTimeVaryingMeasurementNoise1=on  HasMeasurementFcnExtraArgument1=0  HasMeasurementWrapping1=off  MeasurementFcn2=myMeasurementFcn  HasMeasurementJacobianFcn2=off  HasMeasurementEnablePort2=off  HasAdditiveMeasurementNoise2=Additive  MeasurementNoise2=1  HasTimeVaryingMeasurementNoise2=off  HasMeasurementFcnExtraArgument2=0  HasMeasurementWrapping2=off  MeasurementFcn3=myMeasurementFcn  HasMeasurementJacobianFcn3=off  HasMeasurementEnablePort3=off  HasAdditiveMeasurementNoise3=Additive  MeasurementNoise3=1  HasTimeVaryingMeasurementNoise3=off  HasMeasurementFcnExtraArgument3=0  HasMeasurementWrapping3=off  MeasurementFcn4=myMeasurementFcn  HasMeasurementJacobianFcn4=off  HasMeasurementEnablePort4=off  HasAdditiveMeasurementNoise4=Additive  MeasurementNoise4=1  HasTimeVaryingMeasurementNoise4=off  HasMeasurementFcnExtraArgument4=0  HasMeasurementWrapping4=off  MeasurementFcn5=myMeasurementFcn  HasMeasurementJacobianFcn5=off  HasMeasurementEnablePort5=off  HasAdditiveMeasurementNoise5=Additive  MeasurementNoise5=1  HasTimeVaryingMeasurementNoise5=off  HasMeasurementFcnExtraArgument5=0  HasMeasurementWrapping5=off  EnableMultirate=off  StateTransitionFcnSampleTime=1  MeasurementFcn1SampleTime=1  MeasurementFcn2SampleTime=1  MeasurementFcn3SampleTime=1  MeasurementFcn4SampleTime=1  MeasurementFcn5SampleTime=1  UseCurrentEstimator=off  OutputStateCovariance=on  DataType=double  SampleTime=0.001  NumberOfMeasurements=1
  Gain6 : Gain  Gain=1/2/pi
  MATLAB Function : MATLAB Function
  Scope1 : Scope
      settings: ActiveDisplayYMinimum=-1.3479  ActiveDisplayYMaximum=7.13108  DataLoggingVariableName=ScopeData7
  Scope6 : Scope
      settings: ActiveDisplayYMinimum=0.9999988  ActiveDisplayYMaximum=1.0000001
  Selector1 : Selector  InputPortWidth=4  IndexOptions=Index vector (dialog)  Indices=[1]  OutputSizes=1
  Selector8 : Selector  InputPortWidth=4  IndexOptions=Index vector (dialog)  Indices=[3]  OutputSizes=1
  x1hat : Outport
  P : Outport  Port=2
  debug : Outport  Port=3
  xhat_pred : Outport  Port=4
  y_residual : Outport  Port=5
  omega : Outport  Port=6
  wires:
  epsilon/1 -> Extended Kalman Filter1/2
  Constant7/1 -> Extended Kalman Filter1/4
  Constant5/1 -> MATLAB Function/1(gamma)
  Extended Kalman Filter1/2 -> P/1
  y/1 -> Extended Kalman Filter1/3
  MATLAB Function/1(y) -> Extended Kalman Filter1/1
  Extended Kalman Filter1/1 -> Selector1/1, Selector8/1, Scope1/1
  Selector8/1 -> Gain6/1
  Gain6/1 -> omega/1, Scope6/1
  Selector1/1 -> x1hat/1

== system RL_sus_quarter_sim/Quarter_sys/Control/Y_1/IFEKF Select c/Subsystem/MATLAB Function2/IFEKF simple ==
  y : Inport
  Constant : Constant  Value=diag([0,0,0,0,1])
  Constant7 : Constant  Value=10  SampleTime=0.001
  Extended Kalman Filter1 : sharedTrackingLibrary/Extended Kalman Filter  StateTransitionFcn=IFEKF_tfcn_simp  HasStateTransitionJacobianFcn=on  StateTransitionJacobianFcn=IFEKF_jcob_fcn_simp  HasAdditiveProcessNoise=Additive  ProcessNoise=[0,0,1e-7,1e-10,0]  HasTimeVaryingProcessNoise=on  HasStateTransitionFcnExtraArgument=0  InitialState=[0;-1;0;-1;0.1*pi;]  InitialStateCovariance=[1e-1,1e-1,1e-1,1e-1,1e-5]  MeasurementFcn1=IFEKF_measure_fcn_simp  HasMeasurementJacobianFcn1=on  MeasurementJacobianFcn1=IFEKF_mea_jcob_fcn_simp  HasMeasurementEnablePort1=off  HasAdditiveMeasurementNoise1=Additive  MeasurementNoise1=0.0001  HasTimeVaryingMeasurementNoise1=on  HasMeasurementFcnExtraArgument1=0  HasMeasurementWrapping1=off  MeasurementFcn2=myMeasurementFcn  HasMeasurementJacobianFcn2=off  HasMeasurementEnablePort2=off  HasAdditiveMeasurementNoise2=Additive  MeasurementNoise2=1  HasTimeVaryingMeasurementNoise2=off  HasMeasurementFcnExtraArgument2=0  HasMeasurementWrapping2=off  MeasurementFcn3=myMeasurementFcn  HasMeasurementJacobianFcn3=off  HasMeasurementEnablePort3=off  HasAdditiveMeasurementNoise3=Additive  MeasurementNoise3=1  HasTimeVaryingMeasurementNoise3=off  HasMeasurementFcnExtraArgument3=0  HasMeasurementWrapping3=off  MeasurementFcn4=myMeasurementFcn  HasMeasurementJacobianFcn4=off  HasMeasurementEnablePort4=off  HasAdditiveMeasurementNoise4=Additive  MeasurementNoise4=1  HasTimeVaryingMeasurementNoise4=off  HasMeasurementFcnExtraArgument4=0  HasMeasurementWrapping4=off  MeasurementFcn5=myMeasurementFcn  HasMeasurementJacobianFcn5=off  HasMeasurementEnablePort5=off  HasAdditiveMeasurementNoise5=Additive  MeasurementNoise5=1  HasTimeVaryingMeasurementNoise5=off  HasMeasurementFcnExtraArgument5=0  HasMeasurementWrapping5=off  EnableMultirate=off  StateTransitionFcnSampleTime=1  MeasurementFcn1SampleTime=1  MeasurementFcn2SampleTime=1  MeasurementFcn3SampleTime=1  MeasurementFcn4SampleTime=1  MeasurementFcn5SampleTime=1  UseCurrentEstimator=off  OutputStateCovariance=on  DataType=double  SampleTime=0.001  NumberOfMeasurements=1
  Gain6 : Gain  Gain=1/2/pi
  Scope1 : Scope
      settings: ActiveDisplayYMinimum=-108223.31295  ActiveDisplayYMaximum=120159.3313  DataLoggingVariableName=ScopeData2
  Scope6 : Scope
      settings: ActiveDisplayYMinimum=-5.04517  ActiveDisplayYMaximum=3.95687  DataLoggingVariableName=ScopeData3
  Selector1 : Selector  InputPortWidth=5  IndexOptions=Index vector (dialog)  Indices=[1]  OutputSizes=1
  Selector8 : Selector  InputPortWidth=5  IndexOptions=Index vector (dialog)  Indices=[5]  OutputSizes=1
  x1hat : Outport
  P : Outport  Port=2
  debug : Outport  Port=3
  xhat_pred : Outport  Port=4
  y_residual : Outport  Port=5
  omega : Outport  Port=6
  wires:
  y/1 -> Extended Kalman Filter1/2
  Extended Kalman Filter1/2 -> P/1
  Constant7/1 -> Extended Kalman Filter1/3
  Constant/1 -> Extended Kalman Filter1/1
  Gain6/1 -> omega/1, Scope6/1
  Selector8/1 -> Gain6/1
  Selector1/1 -> x1hat/1
  Extended Kalman Filter1/1 -> Selector1/1, Selector8/1, Scope1/1

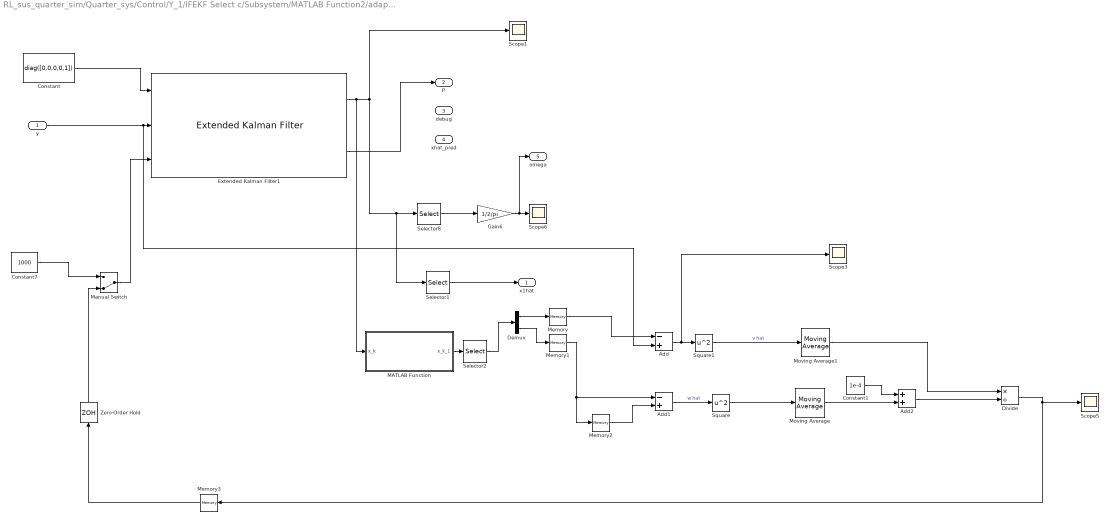
== system RL_sus_quarter_sim/Quarter_sys/Control/Y_1/IFEKF Select c/Subsystem/MATLAB Function2/adaptive IFEKF simple ==
  y : Inport
  Add : Sum  Inputs=-+
  Add1 : Sum  Inputs=-+
  Add2 : Sum
  Constant : Constant  Value=diag([0,0,0,0,1])
  Constant1 : Constant  Value=1e-4
  Constant7 : Constant  Value=1000  SampleTime=0.001
  Demux : Demux  Outputs=2
  Divide : Product  Inputs=*/
  Extended Kalman Filter1 : sharedTrackingLibrary/Extended Kalman Filter  StateTransitionFcn=IFEKF_tfcn_simp  HasStateTransitionJacobianFcn=on  StateTransitionJacobianFcn=IFEKF_jcob_fcn_simp  HasAdditiveProcessNoise=Additive  ProcessNoise=[0,0,1e-7,1e-10,0]  HasTimeVaryingProcessNoise=on  HasStateTransitionFcnExtraArgument=0  InitialState=[0;-1;0;-1;0.1*pi;]  InitialStateCovariance=[1e-1,1e-1,1e-1,1e-1,1e-5]  MeasurementFcn1=IFEKF_measure_fcn_simp  HasMeasurementJacobianFcn1=on  MeasurementJacobianFcn1=IFEKF_mea_jcob_fcn_simp  HasMeasurementEnablePort1=off  HasAdditiveMeasurementNoise1=Additive  MeasurementNoise1=0.0001  HasTimeVaryingMeasurementNoise1=on  HasMeasurementFcnExtraArgument1=0  HasMeasurementWrapping1=off  MeasurementFcn2=myMeasurementFcn  HasMeasurementJacobianFcn2=off  HasMeasurementEnablePort2=off  HasAdditiveMeasurementNoise2=Additive  MeasurementNoise2=1  HasTimeVaryingMeasurementNoise2=off  HasMeasurementFcnExtraArgument2=0  HasMeasurementWrapping2=off  MeasurementFcn3=myMeasurementFcn  HasMeasurementJacobianFcn3=off  HasMeasurementEnablePort3=off  HasAdditiveMeasurementNoise3=Additive  MeasurementNoise3=1  HasTimeVaryingMeasurementNoise3=off  HasMeasurementFcnExtraArgument3=0  HasMeasurementWrapping3=off  MeasurementFcn4=myMeasurementFcn  HasMeasurementJacobianFcn4=off  HasMeasurementEnablePort4=off  HasAdditiveMeasurementNoise4=Additive  MeasurementNoise4=1  HasTimeVaryingMeasurementNoise4=off  HasMeasurementFcnExtraArgument4=0  HasMeasurementWrapping4=off  MeasurementFcn5=myMeasurementFcn  HasMeasurementJacobianFcn5=off  HasMeasurementEnablePort5=off  HasAdditiveMeasurementNoise5=Additive  MeasurementNoise5=1  HasTimeVaryingMeasurementNoise5=off  HasMeasurementFcnExtraArgument5=0  HasMeasurementWrapping5=off  EnableMultirate=off  StateTransitionFcnSampleTime=1  MeasurementFcn1SampleTime=1  MeasurementFcn2SampleTime=1  MeasurementFcn3SampleTime=1  MeasurementFcn4SampleTime=1  MeasurementFcn5SampleTime=1  UseCurrentEstimator=off  OutputStateCovariance=on  DataType=double  SampleTime=0.001  NumberOfMeasurements=1
  Gain6 : Gain  Gain=1/2/pi
  MATLAB Function : MATLAB Function  TreatAsAtomicUnit=on
  Manual Switch : ManualSwitch  CurrentSetting=0
  Memory : Memory  InitialCondition=5
  Memory1 : Memory
  Memory2 : Memory  InitialCondition=1
  Memory3 : Memory  InitialCondition=10
  Moving Average : dspstat3/Moving Average  Method=Exponential weighting  ForgettingFactorPort=off  SpecifyWindowLength=off  WindowLength=100  OverlapLength=50  AllowArbitraryInputLength=on  ForgettingFactor=0.999  SimulateUsing=Interpreted execution
  Moving Average1 : dspstat3/Moving Average  Method=Exponential weighting  ForgettingFactorPort=off  SpecifyWindowLength=off  WindowLength=100  OverlapLength=50  AllowArbitraryInputLength=on  ForgettingFactor=0.999  SimulateUsing=Interpreted execution
  Scope{1,3,5..6} (4 alike) : Scope
      Scope1 settings: ActiveDisplayYMinimum=-108223.31295  ActiveDisplayYMaximum=120159.3313  DataLoggingVariableName=ScopeData3
      Scope3 settings: ActiveDisplayYMinimum=-5.93217  ActiveDisplayYMaximum=3.44712  DataLoggingVariableName=ScopeData4
      Scope5 settings: ActiveDisplayYMinimum=-180.87615  ActiveDisplayYMaximum=1627.8871  DataLoggingVariableName=ScopeData6
      Scope6 settings: ActiveDisplayYMinimum=-2.71822  ActiveDisplayYMaximum=5.24485  DataLoggingVariableName=ScopeData8
  Selector1 : Selector  InputPortWidth=5  IndexOptions=Index vector (dialog)  Indices=[1]  OutputSizes=1
  Selector2 : Selector  InputPortWidth=5  IndexOptions=Index vector (dialog)  Indices=[1 5]  OutputSizes=1
  Selector8 : Selector  InputPortWidth=5  IndexOptions=Index vector (dialog)  Indices=[5]  OutputSizes=1
  Square : Math  Operator=square
  Square1 : Math  Operator=square
  Zero-Order Hold : ZeroOrderHold  SampleTime=0.001
  x1hat : Outport
  P : Outport  Port=2
  debug : Outport  Port=3
  xhat_pred : Outport  Port=4
  omega : Outport  Port=5
  wires:
  Add1/1 -> Square/1  "w hat"
  Demux/2 -> Memory1/1
  Constant1/1 -> Add2/1
  Zero-Order Hold/1 -> Manual Switch/2
  Memory2/1 -> Add1/2
  Manual Switch/1 -> Extended Kalman Filter1/3
  MATLAB Function/1(x_k_1) -> Selector2/1
  Moving Average1/1 -> Divide/1
  Selector2/1 -> Demux/1
  Add2/1 -> Divide/2
  Constant/1 -> Extended Kalman Filter1/1
  Selector1/1 -> x1hat/1
  Moving Average/1 -> Add2/2
  Memory/1 -> Add/1
  Extended Kalman Filter1/1 -> MATLAB Function/1(x_k), Scope1/1, Selector8/1, Selector1/1
  y/1 -> Add/2, Extended Kalman Filter1/2
  Memory1/1 -> Add1/1, Memory2/1
  Square/1 -> Moving Average/1
  Square1/1 -> Moving Average1/1  "v hat"
  Extended Kalman Filter1/2 -> P/1
  Divide/1 -> Memory3/1, Scope5/1
  Selector8/1 -> Gain6/1
  Demux/1 -> Memory/1
  Add/1 -> Scope3/1, Square1/1
  Memory3/1 -> Zero-Order Hold/1
  Gain6/1 -> Scope6/1, omega/1
  Constant7/1 -> Manual Switch/1

== system RL_sus_quarter_sim/Quarter_sys/Control/Y_1/IFEKF Select c/Subsystem2/constant/large C ==
  v_def : Inport
  C : Constant  Value=1500
  Gain : Gain  Gain=-1
  Product1 : Product
  F_sus1 : Outport
  wires:
  v_def/1 -> Product1/1
  Product1/1 -> Gain/1
  Gain/1 -> F_sus1/1
  C/1 -> Product1/2

== system RL_sus_quarter_sim/Quarter_sys/Control/Y_1/IFEKF Select c/Subsystem2/constant/mid C  ==
  v_def : Inport
  Gain : Gain  Gain=-1
  Lmbada_C : Constant  Value=1500
  Product1 : Product
  Out1 : Outport
  wires:
  Product1/1 -> Gain/1
  Lmbada_C/1 -> Product1/2
  v_def/1 -> Product1/1
  Gain/1 -> Out1/1

== system RL_sus_quarter_sim/Quarter_sys/Control/Y_1/IFEKF Select c/Subsystem2/constant/small C ==
  v_def : Inport
  C : Constant  Value=500
  Gain : Gain  Gain=-1
  Product1 : Product
  Out1 : Outport
  wires:
  Gain/1 -> Out1/1
  v_def/1 -> Product1/1
  C/1 -> Product1/2
  Product1/1 -> Gain/1

== system RL_sus_quarter_sim/Quarter_sys/Control/Y_1/IFEKF Select c/Subsystem2/semi ctr/ADD ==
  v_def : Inport
  a_s : Inport  Port=2
  Add : Sum
  Constant7 : Constant  Value=-1
  Constant8 : Constant
  Delta_C : Gain  Gain=500
  Gain : Gain  Gain=-1
  Lmbada_C : Constant  Value=1000
  Product : Product
  Product1 : Product
  Switch : Switch  Criteria=u2 > Threshold  SaturateOnIntegerOverflow=off  InputSameDT=off
  F_sus1 : Outport
  wires:
  Delta_C/1 -> Add/1
  Constant8/1 -> Switch/1
  Add/1 -> Product1/2
  Gain/1 -> F_sus1/1
  Lmbada_C/1 -> Add/2
  Product/1 -> Switch/2
  Product1/1 -> Gain/1
  Switch/1 -> Delta_C/1
  Constant7/1 -> Switch/3
  a_s/1 -> Product/2
  v_def/1 -> Product/1, Product1/1

== system RL_sus_quarter_sim/Quarter_sys/Control/Y_1/IFEKF Select c/Subsystem2/semi ctr/SH ==
  v_def : Inport
  v_s : Inport  Port=2
  Add : Sum
  Constant : Constant  Value=-1
  Constant1 : Constant
  Delta_C : Gain  Gain=500
  Gain : Gain  Gain=-1
  Lmbada_C : Constant  Value=1000
  Product : Product
  Product1 : Product
  Switch : Switch  Criteria=u2 > Threshold  SaturateOnIntegerOverflow=off  InputSameDT=off
  Out1 : Outport
  wires:
  Product/1 -> Switch/2
  Delta_C/1 -> Add/1
  Lmbada_C/1 -> Add/2
  Constant1/1 -> Switch/1
  Product1/1 -> Gain/1
  Add/1 -> Product1/2
  Constant/1 -> Switch/3
  v_def/1 -> Product1/1, Product/1
  Switch/1 -> Delta_C/1
  v_s/1 -> Product/2
  Gain/1 -> Out1/1

== system RL_sus_quarter_sim/Quarter_sys/Control/Y_1/IFEKF Select c/Subsystem2/semi ctr/Subsystem1 ==
  v_def : Inport
  Gain : Gain  Gain=-1
  Lmbada_C : Constant  Value=1500
  Product1 : Product
  Out1 : Outport
  wires:
  Gain/1 -> Out1/1
  v_def/1 -> Product1/1
  Lmbada_C/1 -> Product1/2
  Product1/1 -> Gain/1

== system RL_sus_quarter_sim/Quarter_sys/Control/Y_1/IFEKF freq b/Subsystem/MATLAB Function2/EKF epsilon ==
  y : Inport
  epsilon : Inport  Port=2
  Constant : Constant  Value=diag([0,0,1,0])
  Constant7 : Constant  Value=500  SampleTime=0.001
  Extended Kalman Filter1 : sharedTrackingLibrary/Extended Kalman Filter  StateTransitionFcn=IFEKF_tfcn_ep  HasStateTransitionJacobianFcn=on  StateTransitionJacobianFcn=IFEKF_jcob_fcn_ep  HasAdditiveProcessNoise=Additive  ProcessNoise=[0,0,1e-7,1e-10]  HasTimeVaryingProcessNoise=on  HasStateTransitionFcnExtraArgument=1  InitialState=[0;-0.2;1*2*pi;0.2;]  InitialStateCovariance=[1e-1,1e-1,1e-1,1e-5]  MeasurementFcn1=IFEKF_measure_fcn_mod  HasMeasurementJacobianFcn1=on  MeasurementJacobianFcn1=IFEKF_mea_jcob_fcn_mod  HasMeasurementEnablePort1=off  HasAdditiveMeasurementNoise1=Additive  MeasurementNoise1=0.0001  HasTimeVaryingMeasurementNoise1=on  HasMeasurementFcnExtraArgument1=0  HasMeasurementWrapping1=off  MeasurementFcn2=myMeasurementFcn  HasMeasurementJacobianFcn2=off  HasMeasurementEnablePort2=off  HasAdditiveMeasurementNoise2=Additive  MeasurementNoise2=1  HasTimeVaryingMeasurementNoise2=off  HasMeasurementFcnExtraArgument2=0  HasMeasurementWrapping2=off  MeasurementFcn3=myMeasurementFcn  HasMeasurementJacobianFcn3=off  HasMeasurementEnablePort3=off  HasAdditiveMeasurementNoise3=Additive  MeasurementNoise3=1  HasTimeVaryingMeasurementNoise3=off  HasMeasurementFcnExtraArgument3=0  HasMeasurementWrapping3=off  MeasurementFcn4=myMeasurementFcn  HasMeasurementJacobianFcn4=off  HasMeasurementEnablePort4=off  HasAdditiveMeasurementNoise4=Additive  MeasurementNoise4=1  HasTimeVaryingMeasurementNoise4=off  HasMeasurementFcnExtraArgument4=0  HasMeasurementWrapping4=off  MeasurementFcn5=myMeasurementFcn  HasMeasurementJacobianFcn5=off  HasMeasurementEnablePort5=off  HasAdditiveMeasurementNoise5=Additive  MeasurementNoise5=1  HasTimeVaryingMeasurementNoise5=off  HasMeasurementFcnExtraArgument5=0  HasMeasurementWrapping5=off  EnableMultirate=off  StateTransitionFcnSampleTime=1  MeasurementFcn1SampleTime=1  MeasurementFcn2SampleTime=1  MeasurementFcn3SampleTime=1  MeasurementFcn4SampleTime=1  MeasurementFcn5SampleTime=1  UseCurrentEstimator=off  OutputStateCovariance=on  DataType=double  SampleTime=0.001  NumberOfMeasurements=1
  Gain6 : Gain  Gain=1/2/pi
  Scope6 : Scope
      settings: ActiveDisplayYMinimum=-0.3996  ActiveDisplayYMaximum=6.53697  DataLoggingVariableName=ScopeData2
  Selector1 : Selector  InputPortWidth=4  IndexOptions=Index vector (dialog)  Indices=[1]  OutputSizes=1
  Selector8 : Selector  InputPortWidth=4  IndexOptions=Index vector (dialog)  Indices=[3]  OutputSizes=1
  x1hat : Outport
  P : Outport  Port=2
  debug : Outport  Port=3
  xhat_pred : Outport  Port=4
  y_residual : Outport  Port=5
  omega : Outport  Port=6
  wires:
  y/1 -> Extended Kalman Filter1/3
  Extended Kalman Filter1/2 -> P/1
  Constant7/1 -> Extended Kalman Filter1/4
  epsilon/1 -> Extended Kalman Filter1/2
  Constant/1 -> Extended Kalman Filter1/1
  Gain6/1 -> omega/1, Scope6/1
  Selector8/1 -> Gain6/1
  Extended Kalman Filter1/1 -> Selector1/1, Selector8/1
  Selector1/1 -> x1hat/1

== system RL_sus_quarter_sim/Quarter_sys/Control/Y_1/IFEKF freq b/Subsystem/MATLAB Function2/EKF simple Amp ==
  y : Inport
  epsilon : Inport  Port=2
  Constant5 : Constant  Value=0.1e-5
  Constant7 : Constant  Value=0.11  SampleTime=0.001
  Extended Kalman Filter1 : sharedTrackingLibrary/Extended Kalman Filter  StateTransitionFcn=IFEKF_tfcn_amp  HasStateTransitionJacobianFcn=on  StateTransitionJacobianFcn=IFEKF_jcob_fcn_amp  HasAdditiveProcessNoise=Additive  ProcessNoise=[0,0,1e-7,1e-10]  HasTimeVaryingProcessNoise=on  HasStateTransitionFcnExtraArgument=1  InitialState=[0;-0.5;2*pi;0.5;]  InitialStateCovariance=[1e-1,1e-1,1e-1,1e-5]  MeasurementFcn1=IFEKF_measure_fcn_amp  HasMeasurementJacobianFcn1=on  MeasurementJacobianFcn1=IFEKF_mea_jcob_fcn_amp  HasMeasurementEnablePort1=off  HasAdditiveMeasurementNoise1=Additive  MeasurementNoise1=0.0001  HasTimeVaryingMeasurementNoise1=on  HasMeasurementFcnExtraArgument1=0  HasMeasurementWrapping1=off  MeasurementFcn2=myMeasurementFcn  HasMeasurementJacobianFcn2=off  HasMeasurementEnablePort2=off  HasAdditiveMeasurementNoise2=Additive  MeasurementNoise2=1  HasTimeVaryingMeasurementNoise2=off  HasMeasurementFcnExtraArgument2=0  HasMeasurementWrapping2=off  MeasurementFcn3=myMeasurementFcn  HasMeasurementJacobianFcn3=off  HasMeasurementEnablePort3=off  HasAdditiveMeasurementNoise3=Additive  MeasurementNoise3=1  HasTimeVaryingMeasurementNoise3=off  HasMeasurementFcnExtraArgument3=0  HasMeasurementWrapping3=off  MeasurementFcn4=myMeasurementFcn  HasMeasurementJacobianFcn4=off  HasMeasurementEnablePort4=off  HasAdditiveMeasurementNoise4=Additive  MeasurementNoise4=1  HasTimeVaryingMeasurementNoise4=off  HasMeasurementFcnExtraArgument4=0  HasMeasurementWrapping4=off  MeasurementFcn5=myMeasurementFcn  HasMeasurementJacobianFcn5=off  HasMeasurementEnablePort5=off  HasAdditiveMeasurementNoise5=Additive  MeasurementNoise5=1  HasTimeVaryingMeasurementNoise5=off  HasMeasurementFcnExtraArgument5=0  HasMeasurementWrapping5=off  EnableMultirate=off  StateTransitionFcnSampleTime=1  MeasurementFcn1SampleTime=1  MeasurementFcn2SampleTime=1  MeasurementFcn3SampleTime=1  MeasurementFcn4SampleTime=1  MeasurementFcn5SampleTime=1  UseCurrentEstimator=off  OutputStateCovariance=on  DataType=double  SampleTime=0.001  NumberOfMeasurements=1
  Gain6 : Gain  Gain=1/2/pi
  MATLAB Function : MATLAB Function
  Scope1 : Scope
      settings: ActiveDisplayYMinimum=-1.3479  ActiveDisplayYMaximum=7.13108  DataLoggingVariableName=ScopeData7
  Scope6 : Scope
      settings: ActiveDisplayYMinimum=0.9999988  ActiveDisplayYMaximum=1.0000001
  Selector1 : Selector  InputPortWidth=4  IndexOptions=Index vector (dialog)  Indices=[1]  OutputSizes=1
  Selector8 : Selector  InputPortWidth=4  IndexOptions=Index vector (dialog)  Indices=[3]  OutputSizes=1
  x1hat : Outport
  P : Outport  Port=2
  debug : Outport  Port=3
  xhat_pred : Outport  Port=4
  y_residual : Outport  Port=5
  omega : Outport  Port=6
  wires:
  epsilon/1 -> Extended Kalman Filter1/2
  Constant7/1 -> Extended Kalman Filter1/4
  Constant5/1 -> MATLAB Function/1(gamma)
  Extended Kalman Filter1/2 -> P/1
  y/1 -> Extended Kalman Filter1/3
  MATLAB Function/1(y) -> Extended Kalman Filter1/1
  Extended Kalman Filter1/1 -> Selector1/1, Selector8/1, Scope1/1
  Selector8/1 -> Gain6/1
  Gain6/1 -> omega/1, Scope6/1
  Selector1/1 -> x1hat/1
